simulink model "Lab_1_Anti_WindUp"  (R2022a)
settings: Solver=VariableStepAuto  StartTime=0.0  StopTime=50  RelTol=1e-3
values from neighbouring files (symbols this model uses):
  y = num(1)/den(1)    [Lab_1.m]
undefined symbols (not defined in the file or in its folder): den1, num1
settings Model: Creator=pdidd  LastModifiedBy=pdidd

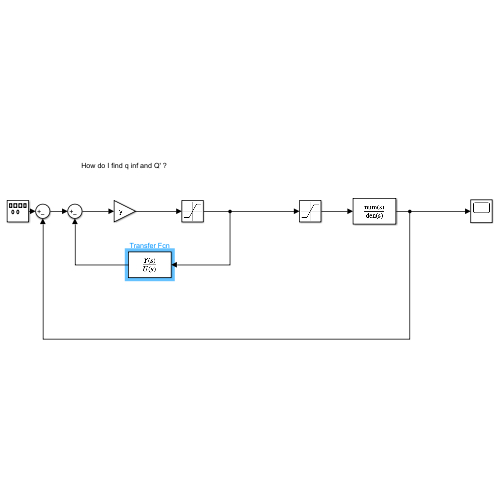
[thumbnail: Simulink's stored preview of the top-level diagram]
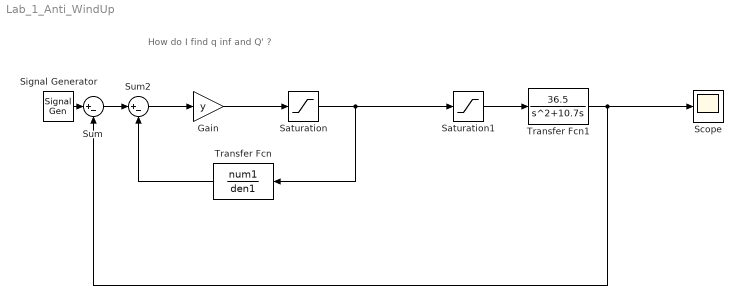
== system Lab_1_Anti_WindUp ==
  note: How do I find q inf and Q' ?
  Gain : Gain  Gain=y
  Saturation : Saturate  UpperLimit=10  LowerLimit=-10
  Saturation1 : Saturate  UpperLimit=10  LowerLimit=-10
  Scope : Scope
  Signal Generator : SignalGenerator  WaveForm=square  Amplitude=2.5  Frequency=0.4  Units=rad/sec
  Sum : Sum  Inputs=|+-
  Sum2 : Sum  Inputs=|+-
  Transfer Fcn : TransferFcn  Numerator=num1  Denominator=den1
  Transfer Fcn1 : TransferFcn  Numerator=[36.5]  Denominator=[1 10.7 0]
  wires:
  Signal Generator/1 -> Sum/1
  Saturation/1 -> Transfer Fcn/1, Saturation1/1
  Saturation1/1 -> Transfer Fcn1/1
  Transfer Fcn1/1 -> Sum/2, Scope/1
  Gain/1 -> Saturation/1
  Transfer Fcn/1 -> Sum2/2
  Sum/1 -> Sum2/1
  Sum2/1 -> Gain/1
